simulink model "inv_pen_simulink"  (R2020b)
settings: Solver=VariableStepAuto  StartTime=0.0  StopTime=10.0  RelTol=1e-3
values from neighbouring files (symbols this model uses):
  k = lqr(A, B, Q, R)    [params.m]
  theta_d_init = 0    [params.m]
  theta_init = 0.01    [params.m]
  x_d_init = 0    [params.m]
  x_init = 0    [params.m]
settings Model: Creator=Admin  LastModifiedBy=Admin

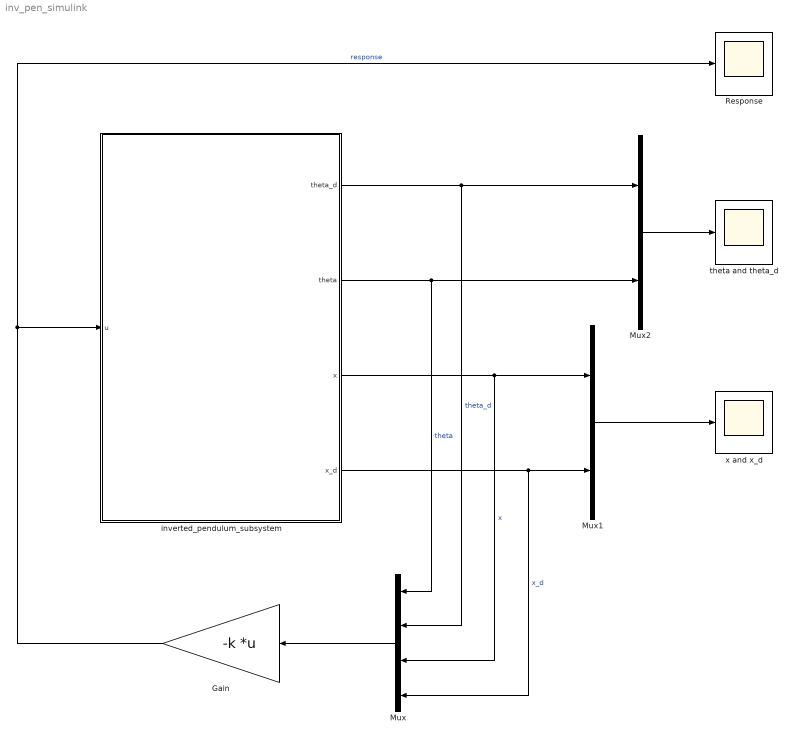
== system inv_pen_simulink ==
  Gain : Gain  Gain=-k  Multiplication=Matrix(K*u) (u vector)
  Mux : Mux
  Mux1 : Mux  Inputs=2
  Mux2 : Mux  Inputs=2
  Response : Scope
  inverted_pendulum_subsystem : Subsystem
  theta and theta_d : Scope
  x and x_d : Scope
  wires:
  inverted_pendulum_subsystem/3(x) -> Mux/3, Mux1/1  "x"
  inverted_pendulum_subsystem/4(x_d) -> Mux/4, Mux1/2  "x_d"
  inverted_pendulum_subsystem/1(theta_d) -> Mux/2, Mux2/1  "theta_d"
  inverted_pendulum_subsystem/2(theta) -> Mux/1, Mux2/2  "theta"
  Mux2/1 -> theta and theta_d/1
  Mux1/1 -> x and x_d/1
  Mux/1 -> Gain/1
  Gain/1 -> Response/1, inverted_pendulum_subsystem/1(u)  "response"

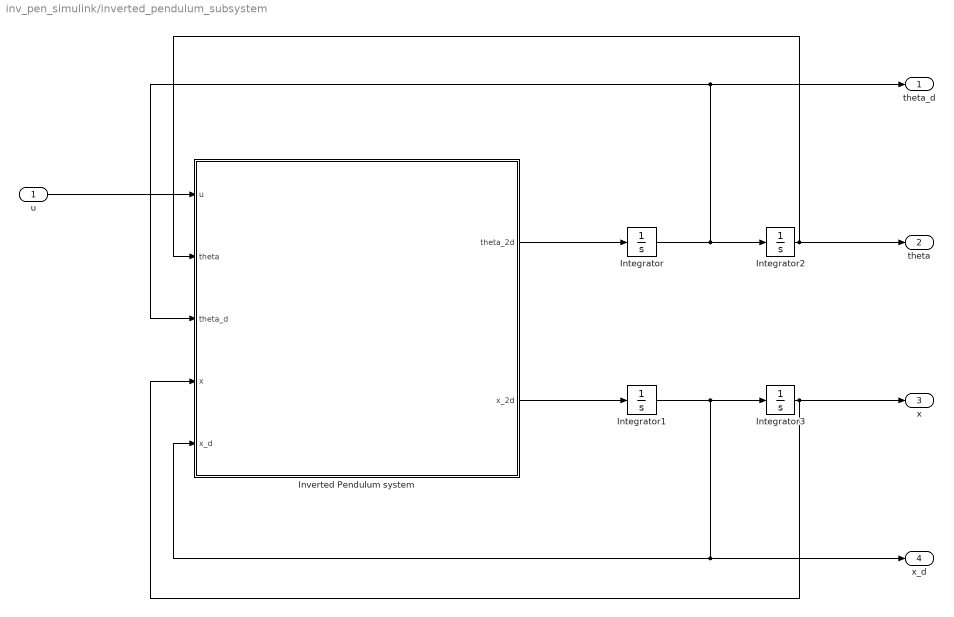
== system inv_pen_simulink/inverted_pendulum_subsystem ==
  u : Inport
  Integrator : Integrator  InitialCondition=theta_d_init
  Integrator1 : Integrator  InitialCondition=x_d_init
  Integrator2 : Integrator  InitialCondition=theta_init
  Integrator3 : Integrator  InitialCondition=x_init
  Inverted Pendulum system : MATLAB Function  TreatAsAtomicUnit=on
  theta_d : Outport
  theta : Outport  Port=2
  x : Outport  Port=3
  x_d : Outport  Port=4
  wires:
  Integrator/1 -> theta_d/1, Inverted Pendulum system/3(theta_d), Integrator2/1
  Integrator3/1 -> x/1, Inverted Pendulum system/4(x)
  Integrator1/1 -> x_d/1, Inverted Pendulum system/5(x_d), Integrator3/1
  u/1 -> Inverted Pendulum system/1(u)
  Integrator2/1 -> theta/1, Inverted Pendulum system/2(theta)
  Inverted Pendulum system/1(theta_2d) -> Integrator/1
  Inverted Pendulum system/2(x_2d) -> Integrator1/1

== matlab function inv_pen_simulink/inverted_pendulum_subsystem/Inverted Pendulum system ==
  data: u input; theta_2d output; theta input; theta_d input; x input; x_d input; x_2d output
function [theta_2d, x_2d] = Inverted_Pendulum(u, theta, theta_d, x, x_d)
% Simulink model for inverted pendulum system

% System parameters
M = 1;      % Mass of the cart (kg)
m = 0.1;    % Mass of the pendulum (kg)
l = 1;      % Length of the pendulum rod (m)
g = 9.81;   % Gravitational acceleration (m/s^2)

x_2d = (u + m*l*sin(theta)*(theta_d)^2 - m*g*cos(theta)*sin(theta)) / ...
       (M + m - m*(cos(theta))^2);

theta_2d = (u*cos(theta) - (M + m)*g*sin(theta) + ...
           m*l*cos(theta)*sin(theta)*(theta_d)^2) / ...
           (m*l*(cos(theta))^2 - (M + m)*l);
end
